simulink model "Simple_Preisach"  (R2017b)
settings: Solver=FixedStepAuto  StartTime=0.0  StopTime=simTotalTime  FixedStep=0.05  MaxStep=0.1  MinStep=0.01  RelTol=1e-3
undefined symbols (not defined in the file): gridArea, gridDen, gridLength, hysteronMax, hysteronMin, initialInput, initialRelays, inputFactor, inputMax, inputMin, offset, outputFactor, outputMax, outputMin, simTotalTime, weightFunc, xyGrid
libraries: simulink x1
settings Model: Creator=Marco  LastModifiedBy=M. Vasquez Beltran

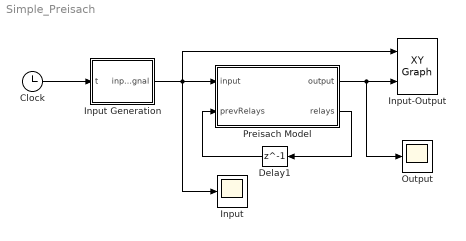
== system Simple_Preisach ==
  Clock : Clock
  Delay1 : Delay  DelayLength=1  InitialCondition=initialRelays
  Input : Scope
  Input Generation : MATLAB Function  TreatAsAtomicUnit=on
  Input-Output : simulink/Sinks/XY Graph  xmin=inputMin*inputFactor  xmax=inputMax*inputFactor  ymin=outputMin*outputFactor  ymax=outputMax*outputFactor  st=-1
  Output : Scope
  Preisach Model : MATLAB Function  TreatAsAtomicUnit=on
  wires:
  Preisach Model/2(relays) -> Delay1/1
  Delay1/1 -> Preisach Model/2(prevRelays)
  Clock/1 -> Input Generation/1(t)
  Input Generation/1(inputSignal) -> Input/1, Input-Output/1, Preisach Model/1(input)
  Preisach Model/1(output) -> Output/1, Input-Output/2

== matlab function Simple_Preisach/Input Generation ==
  data: t input; simTotalTime parameter; inputSignal output; inputMin parameter; inputMax parameter; initialInput parameter
function inputSignal = fcn(t,...
    simTotalTime, inputMin, inputMax, initialInput)

inputMinFactor = 1.00;
inputMaxFactor = 1.00;

% amplitude = (inputMaxFactor*inputMax - inputMinFactor*inputMin)/2;

% timeFactor = ( simTotalTime - 1.0*t )/simTotalTime;
% amplitude = timeFactor*(inputMaxFactor*inputMax - inputMinFactor*inputMin)/2;

divTime = simTotalTime/4.11;
if(t<divTime)
    timeFactor = 1 - 1.0*t/divTime;
else
    timeFactor = 1.0*(t - divTime)/(simTotalTime - divTime);
end
amplitude = timeFactor*(inputMaxFactor*inputMax - inputMinFactor*inputMin)/2;

offset = (inputMaxFactor*inputMax + inputMinFactor*inputMin)/2;
freq = 1/40;
% phase = -asin((initialInput - offset)/amplitude);

% amplitude = 3;
% offset = -3;
% freq = 1/40;
phase = 0;

inputSignal = amplitude * sin( 2*pi*freq*t - phase ) + offset;

== matlab function Simple_Preisach/Preisach Model ==
  data: input input; prevRelays input; output output; weightFunc parameter; relays output; offset parameter; hysteronMin parameter; hysteronMax parameter; gridDen parameter; xyGrid parameter; gridLength parameter; gridArea parameter
function [output, relays] = fcn(input, prevRelays, ...
    weightFunc, offset, hysteronMin, hysteronMax, gridDen, xyGrid, gridLength, gridArea)

%     output = offset;
%     relays = prevRelays;
%     for i=1:gridDen
%         ii = gridDen-i+1; %index inversion for rows
%         for j=1:i
%             if( input >= xyGrid(i) && relays(ii,j) ~= hysteronMax )
%                 relays(ii,j) = hysteronMax;
%             elseif( input <= xyGrid(j) && relays(ii,j) ~= hysteronMin )
%                 relays(ii,j) = hysteronMin;
%             end
%             output = output + relays(ii,j)*weightFunc(ii,j)*gridArea;
%         end
%     end



%     relays = prevRelays;
%     for row=1:gridDen+1
%         if( row == gridDen+1 || input <= xyGrid(row) )
%             row = row-1;
%             irow = gridDen-row+1;
%             relays(irow:end, 1:row) = hysteronMax*fliplr(triu(ones(row, row)));
%             break;
%         end
%     end
%     for col=gridDen:-1:0
%         if( col == 0 || input >= xyGrid(col) )
%             col = col+1;
%             irow = gridDen-col+1;
%             relays(1:irow, col:end) = hysteronMin*fliplr(triu(ones(irow, irow)));
%             break;
%         end
%     end
%     output = sum(sum(relays(:,:).*weightFunc(:,:)))*gridArea + offset;



    relays = prevRelays;
    if( xyGrid(end) <= input )
        relays(:,:) = hysteronMax*fliplr(triu(ones(gridDen, gridDen)));
    elseif( input < xyGrid(1) )
        relays(:,:) = hysteronMin*fliplr(triu(ones(gridDen, gridDen)));
    else
        idx0 = 1;
        while( idx0 <= gridDen-1 )
            if( xyGrid(idx0) <= input && input < xyGrid(idx0+1) )
                col = idx0;
                row = gridDen-idx0+1;

                relays(row:end, 1:col) = hysteronMax*fliplr(triu(ones(col, col)));
                relays(1:row-1, col+1:end) = hysteronMin*fliplr(triu(ones(row-1, row-1)));
                break;
            end
            idx0 = idx0 + 1;
        end
    end
    output = sum(sum(relays(:,:).*weightFunc(:,:)))*gridArea + offset;
